simulink model "firstharmonic"  (R2024a)
settings: Solver=VariableStepAuto  StartTime=0.0  StopTime=10.0  RelTol=1e-3
values from neighbouring files (symbols this model uses):
  b = b_values(i)    [firstharmonicbodeplots.m]    (also in stabilitycriterions.m = -0.5; untitled.m)
settings Model: Creator=Hp  LastModifiedBy=Hp

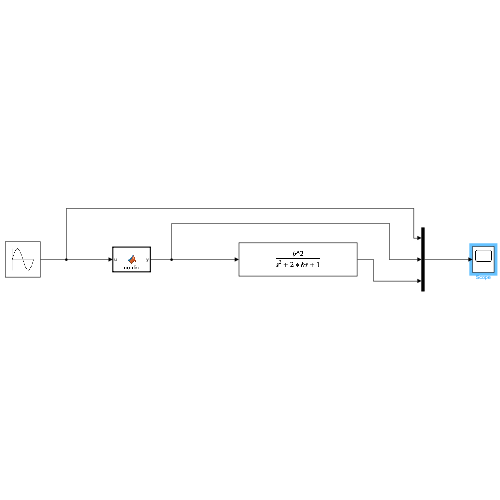
[thumbnail: Simulink's stored preview of the top-level diagram]
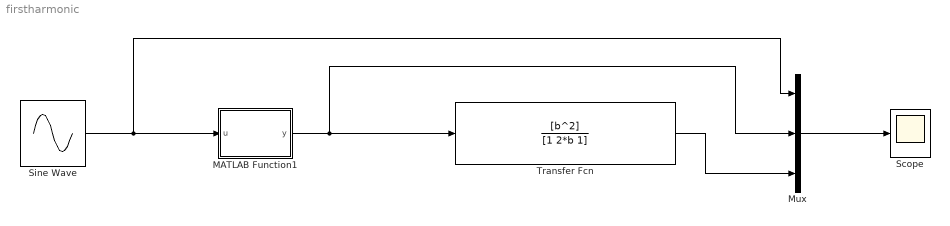
== system firstharmonic ==
  MATLAB Function1 : MATLAB Function  TreatAsAtomicUnit=on
  Mux : Mux  Inputs=3
  Scope : Scope
  Sine Wave : Sin  Frequency=5  SampleTime=0
  Transfer Fcn : TransferFcn  Numerator=[b^2]  Denominator=[1 2*b 1]
  wires:
  Mux/1 -> Scope/1
  MATLAB Function1/1(y) -> Mux/2, Transfer Fcn/1
  Sine Wave/1 -> MATLAB Function1/1(u), Mux/1
  Transfer Fcn/1 -> Mux/3

== matlab function firstharmonic/MATLAB Function1 ==
  data: u input; y output
function y = nonlin(u)
k=2;
a=1;
    if u > a
        y = k*a;      % saturate at +k*a
    elseif u < -a
        y = -k*a;     % saturate at -k*a
    else
        y = k*u;      % linear region
    end
end
